simulink model "assign1_2"  (R2020b)
settings: Solver=ode3  StartTime=0.0  StopTime=500  FixedStep=0.01  MinStep=0.01  RelTol=1e-3
settings Model: Creator=10911  LastModifiedBy=10911

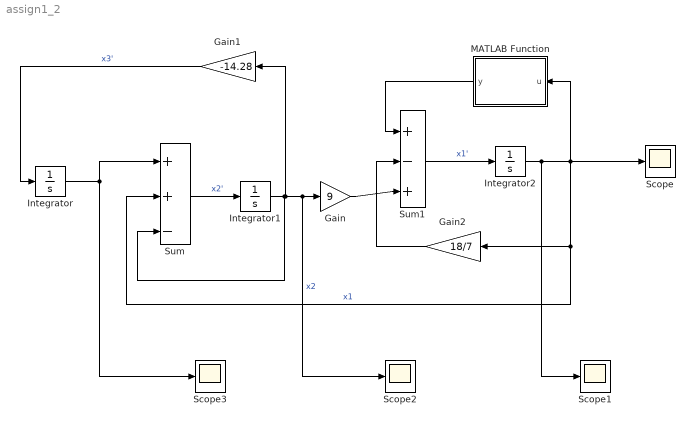
== system assign1_2 ==
  Gain : Gain  Gain=9
  Gain1 : Gain  Gain=-14.28
  Gain2 : Gain  Gain=18/7
  Integrator : Integrator  InitialCondition=3
  Integrator1 : Integrator  InitialCondition=2
  Integrator2 : Integrator  InitialCondition=1
  MATLAB Function : MATLAB Function  TreatAsAtomicUnit=on
  Scope{,1..3} (4 alike) : Scope
  Sum : Sum  Inputs=|++-
  Sum1 : Sum  Inputs=|+-+
  wires:
  Integrator1/1 -> Sum/3, Scope2/1, Gain/1, Gain1/1  "x2"
  Gain1/1 -> Integrator/1  "x3'"
  Integrator/1 -> Scope3/1, Sum/1
  Sum/1 -> Integrator1/1  "x2'"
  Sum1/1 -> Integrator2/1  "x1'"
  Gain/1 -> Sum1/3
  Integrator2/1 -> Scope1/1, MATLAB Function/1(u), Scope/1, Gain2/1, Sum/2  "x1"
  Gain2/1 -> Sum1/2
  MATLAB Function/1(y) -> Sum1/1

== matlab function assign1_2/MATLAB Function ==
  data: u input; y output
function y = fcn(u)

y = 9*3/14*(abs(u+1)-abs(u-1));
